simulink model "simulateur_1"  (R2022b)
settings: Solver=FixedStepAuto  StartTime=0.0  StopTime=10.0  FixedStep=dt  RelTol=1e-3
model workspace: external: MATLAB File /Users/antoine/Desktop/GPH/H2023/Design_2/simulation_équipe_1/init.m (data not in the file)
values from neighbouring files (symbols this model uses):
  dt = 0.000125    [init.m]
  f_1 = 100    [init.m]
  mode = 2    [init.m]
undefined symbols (not defined in the file or in its folder): magnitude
libraries: simulink x1, slpidlib x1, dspstat3 x1
settings Model: Creator=antoine  LastModifiedBy=antoine

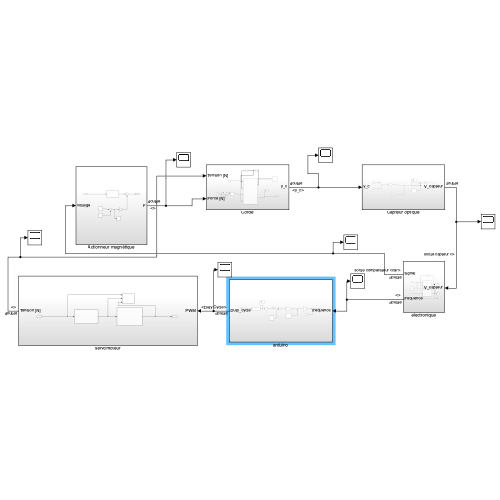
[thumbnail: Simulink's stored preview of the top-level diagram]
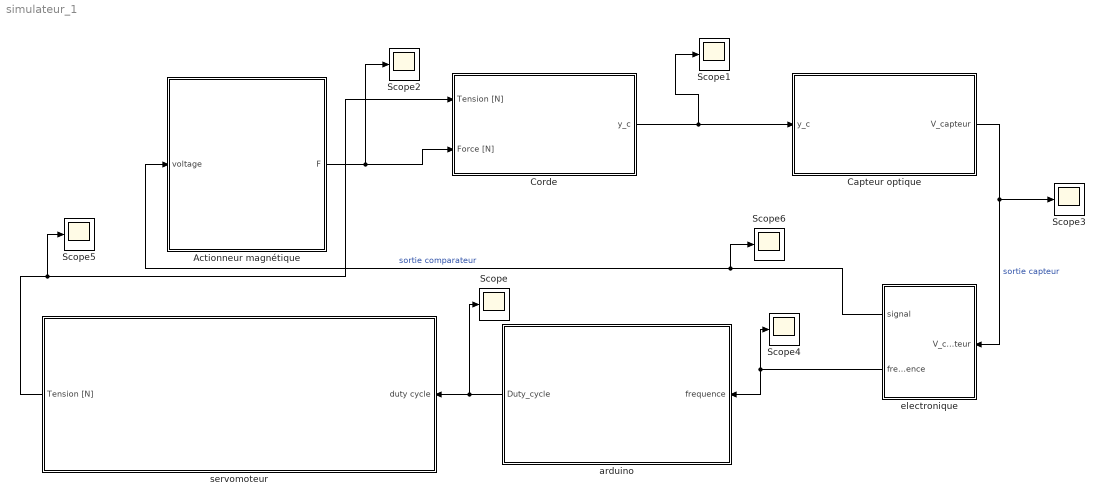
== system simulateur_1 ==
  Actionneur magnétique : Subsystem
  Capteur optique : Subsystem
  Corde : Subsystem
  Scope{,1..6} (7 alike) : Scope
  arduino : Subsystem
  electronique : Subsystem
  servomoteur : Subsystem
  wires:
  Corde/1(y_c) -> Capteur optique/1(y_c), Scope1/1
  Capteur optique/1(V_capteur) -> Scope3/1, electronique/1(V_capteur)  "sortie capteur"
  servomoteur/1(Tension [N]) -> Corde/1(Tension [N]), Scope5/1
  Actionneur magnétique/1(F) -> Scope2/1, Corde/2(Force [N])
  electronique/1(signal) -> Scope6/1, Actionneur magnétique/1(voltage)  "sortie comparateur"
  electronique/2(frequence) -> arduino/1(frequence), Scope4/1
  arduino/1(Duty_cycle) -> Scope/1, servomoteur/1(duty cycle)

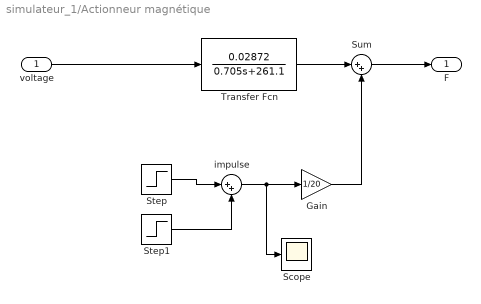
== system simulateur_1/Actionneur magnétique ==
  voltage : Inport
  Gain : Gain  Gain=1/20
  Scope : Scope
  Step : Step  Time=3*dt  SampleTime=0
  Step1 : Step  Time=6*dt  After=-1  SampleTime=0
  Sum : Sum  Inputs=|++
  Transfer Fcn : TransferFcn  Numerator=[0.02872]  Denominator=[0.705 261.1]
  impulse : Sum  Inputs=|++
  F : Outport
  wires:
  voltage/1 -> Transfer Fcn/1
  Transfer Fcn/1 -> Sum/1
  Sum/1 -> F/1
  Gain/1 -> Sum/2
  Step/1 -> impulse/1
  Step1/1 -> impulse/2
  impulse/1 -> Scope/1, Gain/1

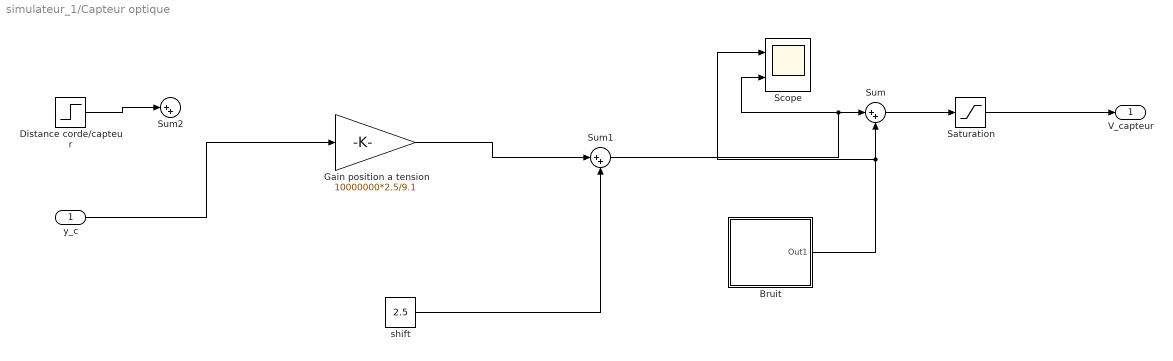
== system simulateur_1/Capteur optique ==
  y_c : Inport
  Bruit : Subsystem
  "Distance corde/capteur " : Step  Time=dt  After=0.00381  SampleTime=0
  Gain position a tension : Gain  Gain=10000000*2.5/9.1
  Saturation : Saturate  UpperLimit=5  LowerLimit=0
  Scope : Scope  NumInputPorts=2
  Sum : Sum  Inputs=|++
  Sum1 : Sum  Inputs=|++
  Sum2 : Sum  Inputs=|++
  shift : Constant  Value=2.5
  V_capteur : Outport
  wires:
  Sum/1 -> Saturation/1
  shift/1 -> Sum1/2
  Gain position a tension/1 -> Sum1/1
  Sum1/1 -> Scope/2, Sum/1
  Bruit/1(Out1) -> Scope/1, Sum/2
  Saturation/1 -> V_capteur/1
  "Distance corde/capteur "/1 -> Sum2/1
  y_c/1 -> Gain position a tension/1

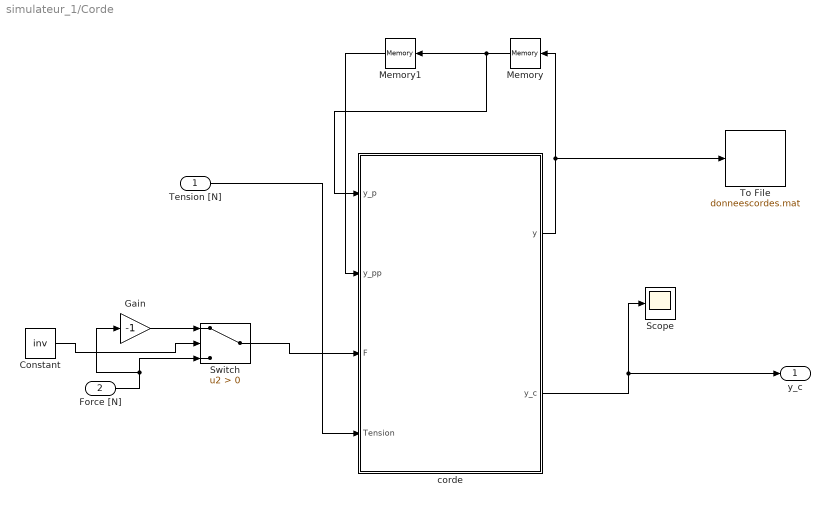
== system simulateur_1/Corde ==
  Tension [N] : Inport
  Force [N] : Inport  Port=2
  Constant : Constant  Value=inv
  Gain : Gain  Gain=-1
  Memory : Memory
  Memory1 : Memory
  Scope : Scope
  Switch : Switch  Criteria=u2 > Threshold  SaturateOnIntegerOverflow=off  InputSameDT=off
  To File : ToFile  Filename=donneescordes.mat  SaveFormat=Timeseries
  corde : MATLAB Function  TreatAsAtomicUnit=on
  y_c : Outport
  wires:
  corde/2(y_c) -> Scope/1, y_c/1
  Memory/1 -> corde/1(y_p), Memory1/1
  Memory1/1 -> corde/2(y_pp)
  corde/1(y) -> Memory/1, To File/1
  Switch/1 -> corde/3(F)
  Gain/1 -> Switch/1
  Force [N]/1 -> Switch/3, Gain/1
  Constant/1 -> Switch/2
  Tension [N]/1 -> corde/4(Tension)

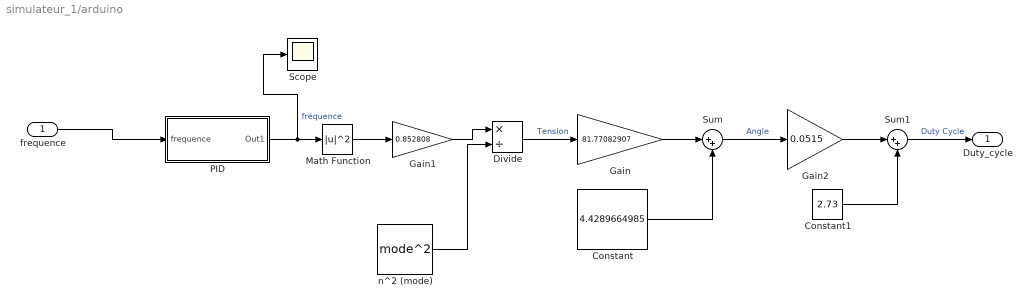
== system simulateur_1/arduino ==
  frequence : Inport
  Constant : Constant  Value=4.4289664985
  Constant1 : Constant  Value=2.73
  Divide : Product  Inputs=*/
  Gain : Gain  Gain=81.77082907
  Gain1 : Gain  Gain=0.852808
  Gain2 : Gain  Gain=0.0515
  Math Function : Math  Operator=magnitude^2
  PID : Subsystem
  Scope : Scope
  Sum : Sum  Inputs=|++
  Sum1 : Sum  Inputs=|++
  n^2 (mode) : Constant  Value=mode^2
  Duty_cycle : Outport
  wires:
  n^2 (mode)/1 -> Divide/2
  Gain1/1 -> Divide/1
  Gain2/1 -> Sum1/1
  Constant1/1 -> Sum1/2
  Divide/1 -> Gain/1  "Tension"
  Math Function/1 -> Gain1/1
  Gain/1 -> Sum/1
  PID/1(Out1) -> Scope/1, Math Function/1  "fréquence"
  Constant/1 -> Sum/2
  Sum1/1 -> Duty_cycle/1  "Duty Cycle"
  Sum/1 -> Gain2/1  "Angle"
  frequence/1 -> PID/1(frequence)

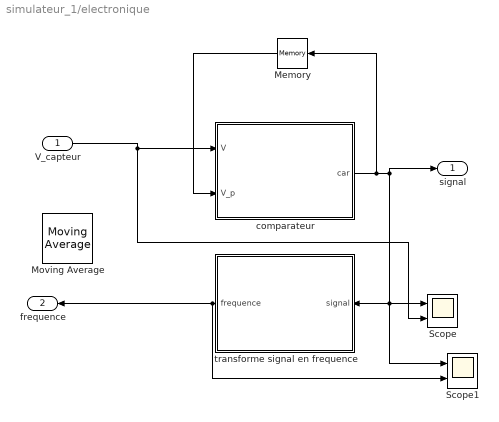
== system simulateur_1/electronique ==
  V_capteur : Inport
  Memory : Memory
  Moving Average : dspstat3/Moving Average  Method=Sliding window  ForgettingFactorPort=off  SpecifyWindowLength=on  WindowLength=10  OverlapLength=9  AllowArbitraryInputLength=off  ForgettingFactor=0.99  SimulateUsing=Interpreted execution
  Scope : Scope  NumInputPorts=2
  Scope1 : Scope  NumInputPorts=2
  comparateur : MATLAB Function  TreatAsAtomicUnit=on
  transforme signal en frequence : Subsystem
  signal : Outport
  frequence : Outport  Port=2
  wires:
  comparateur/1(car) -> Scope1/1, transforme signal en frequence/1(signal), Scope/1, signal/1, Memory/1
  Memory/1 -> comparateur/2(V_p)
  V_capteur/1 -> Scope/2, comparateur/1(V)
  transforme signal en frequence/1(frequence) -> Scope1/2, frequence/1

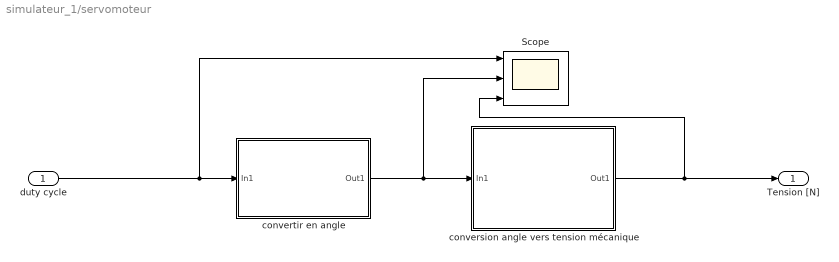
== system simulateur_1/servomoteur ==
  duty cycle : Inport
  Scope : Scope  NumInputPorts=3
  conversion angle vers tension mécanique : Subsystem
  convertir en angle : Subsystem
  Tension [N] : Outport
  wires:
  duty cycle/1 -> Scope/1, convertir en angle/1(In1)
  convertir en angle/1(Out1) -> Scope/2, conversion angle vers tension mécanique/1(In1)
  conversion angle vers tension mécanique/1(Out1) -> Scope/3, Tension [N]/1

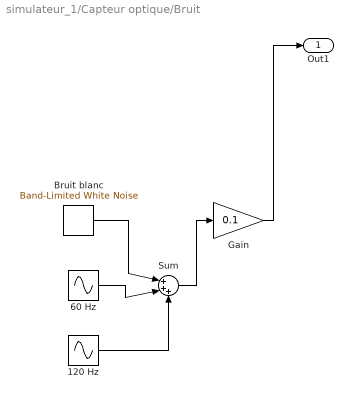
== system simulateur_1/Capteur optique/Bruit ==
  120 Hz : Sin  Frequency=120  SampleTime=0
  60 Hz : Sin  Frequency=60  SampleTime=0
  Bruit blanc : simulink/Sources/Band-Limited White Noise  Cov=[0.1]  Ts=0.1  seed=[23341]
  Gain : Gain  Gain=0.1
  Sum : Sum  Inputs=|+++
  Out1 : Outport
  wires:
  Bruit blanc/1 -> Sum/1
  60 Hz/1 -> Sum/2
  120 Hz/1 -> Sum/3
  Sum/1 -> Gain/1
  Gain/1 -> Out1/1

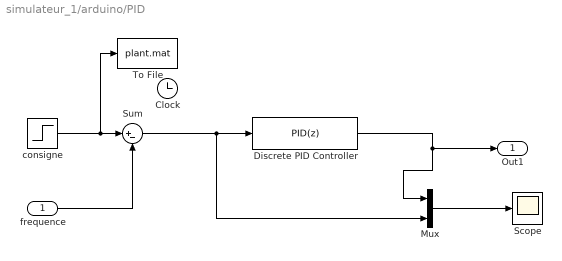
== system simulateur_1/arduino/PID ==
  frequence : Inport
  Clock : Clock
  Discrete PID Controller : slpidlib/PID Controller  Controller=PID  Form=Ideal  TimeDomain=Discrete-time  UseExternalTs=off  SampleTime=-1  IntegratorMethod=Trapezoidal  FilterMethod=Trapezoidal  ControllerParametersSource=internal  P=0.5  I=4.1  UseKiTs=off  D=0.4  N=10  UseFilter=on  TunerSelectOption=Transfer Function Based (PID Tuner App)  InitialConditionSource=internal  InitialConditionForIntegrator=0  InitialConditionForFilter=0  DifferentiatorICPrevScaledInput=0  ExternalReset=none  TrackingMode=off  Kt=1  LimitOutput=on  SatLimitsSource=internal  UpperSaturationLimit=1000  LowerSaturationLimit=-1000  LinearizeAsGain=off  AntiWindupMode=clamping  Kb=1  LimitIntegrator=on  UpperIntegratorSaturationLimit=1000  LowerIntegratorSaturationLimit=-1000  POutMin=[-1000]  POutMax=[1000]  IOutMin=[-1000]  IOutMax=[1000]  DOutMin=[-1000]  DOutMax=[1000]  NOutMin=[-1000]  NOutMax=[1000]  SumOutMin=[-1000]  SumOutMax=[1000]  SaturationOutMin=[]  SaturationOutMax=[]  PParamMin=[]  PParamMax=[]  IParamMin=[]  IParamMax=[]  DParamMin=[]  DParamMax=[]  NParamMin=[]  NParamMax=[]  KbParamMin=[]  KbParamMax=[]  KtParamMin=[]  KtParamMax=[]  KbOutMin=[]  KbOutMax=[]  KtOutMin=[]  KtOutMax=[]  IntegratorOutMin=[]  IntegratorOutMax=[]  FilterOutMin=[]  FilterOutMax=[]  SumI1OutMin=[]  SumI1OutMax=[]  SumI2OutMin=[]  SumI2OutMax=[]  SumI3OutMin=[]  SumI3OutMax=[]  SumI4OutMin=[]  SumI4OutMax=[]  SumDOutMin=[]  SumDOutMax=[]  DifferentiatorOutMin=[]  DifferentiatorOutMax=[]  FilterDiffOutCoefMin=[]  FilterDiffOutCoefMax=[]  ReciprocalOutMin=[]  ReciprocalOutMax=[]  SumDenOutMin=[]  SumDenOutMax=[]  SumNumOutMin=[]  SumNumOutMax=[]  DivideOutMin=[]  DivideOutMax=[]  UdiffTsProdOutMin=[]  UdiffTsProdOutMax=[]  NTsProdOutMin=[]  NTsProdOutMax=[]  UintegralTsProdOutMin=[]  UintegralTsProdOutMax=[]  UngainTsProdOutMin=[]  UngainTsProdOutMax=[]  ClampingZeroOutDataTypeStr=Inherit: Inherit via back propagation  ClampingZeroOutMin=[]  ClampingZeroOutMax=[]  FilterDenConstantOutDataTypeStr=Inherit: Inherit via back propagation  FilterDenConstantOutMin=[]  FilterDenConstantOutMax=[]  PCopyOutDataTypeStr=Inherit: Inherit via back propagation  PCopyOutMin=[]  PCopyOutMax=[]  NCopyOutDataTypeStr=Inherit: Inherit via back propagation  NCopyOutMin=[]  NCopyOutMax=[]  IntegratorContinuousStateAttributes=''  IntegratorStateMustResolveToSignalObject=off  IntegratorRTWStateStorageClass=Auto  FilterContinuousStateAttributes=''  FilterStateMustResolveToSignalObject=off  FilterRTWStateStorageClass=Auto  ParallelPVariant=Passthrough  IdealPVariant=InternalParameters  IVariant=InternalParameters  DVariant=InternalParameters  IntegratorVariant=Discrete  SatVariant=Enabled  AWVariant=DiscClampingIdeal  PCopyVariant=InternalParamsIdeal  TRVariant=Disabled  FdbkBlocksVariant=Feedback  IdealPFdbkVariant=InternalParameters  SatFdbkVariant=Passthrough  DerivativeFilterVariant=TrapezoidalFilter  NVariant=InternalParameters  NCopyVariant=InternalParameters  FilterICVariant=InternalICsFilter  IntegratorICVariant=InternalICs  ExternalResetVariant=Disabled  TRSumVariant=Passthrough  SumFdbkVariant=Enabled  SumVariant=Sum_PID  TsampFilterVariant=InternalTs  TsampNgainVariant=Passthrough  TsampIntegralVariant=Passthrough  ExternalSaturationOutDataTypeStr=Inherit: Same as second input
      settings: LibrarySourceBlock=simulink/Discrete/Discrete PID Controller
  Mux : Mux  Inputs=2
  Scope : Scope
  Sum : Sum  Inputs=|+-
  To File : ToFile  Filename=plant.mat  SaveFormat=Timeseries
  consigne : Step  Time=0  After=f_1  SampleTime=10
  Out1 : Outport
  wires:
  Mux/1 -> Scope/1
  consigne/1 -> To File/1, Sum/1
  frequence/1 -> Sum/2
  Sum/1 -> Discrete PID Controller/1, Mux/2
  Discrete PID Controller/1 -> Mux/1, Out1/1

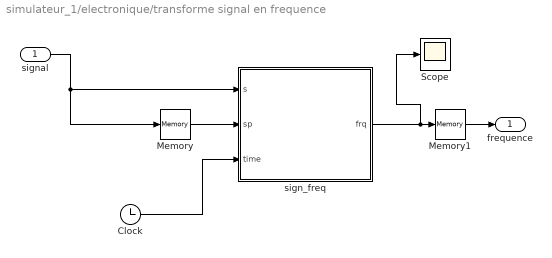
== system simulateur_1/electronique/transforme signal en frequence ==
  signal : Inport
  Clock : Clock
  Memory : Memory  InitialCondition=5
  Memory1 : Memory  InitialCondition=100
  Scope : Scope
  sign_freq : MATLAB Function  TreatAsAtomicUnit=on
  frequence : Outport
  wires:
  signal/1 -> Memory/1, sign_freq/1(s)
  sign_freq/1(frq) -> Memory1/1, Scope/1
  Clock/1 -> sign_freq/3(time)
  Memory/1 -> sign_freq/2(sp)
  Memory1/1 -> frequence/1

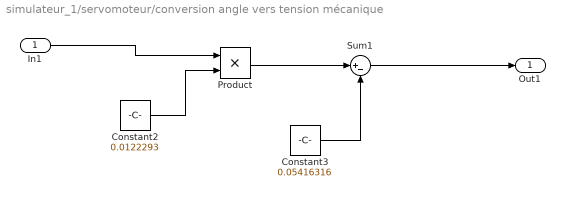
== system simulateur_1/servomoteur/conversion angle vers tension mécanique ==
  In1 : Inport
  Constant2 : Constant  Value=0.0122293
  Constant3 : Constant  Value=0.05416316
  Product : Product
  Sum1 : Sum  Inputs=|+-
  Out1 : Outport
  wires:
  Constant2/1 -> Product/2
  In1/1 -> Product/1
  Sum1/1 -> Out1/1
  Product/1 -> Sum1/1
  Constant3/1 -> Sum1/2

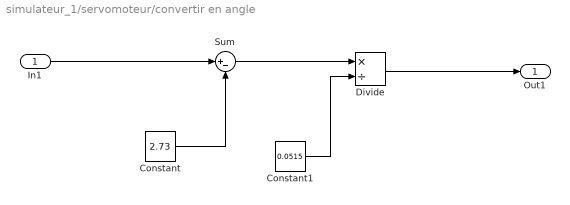
== system simulateur_1/servomoteur/convertir en angle ==
  In1 : Inport
  Constant : Constant  Value=2.73
  Constant1 : Constant  Value=0.0515
  Divide : Product  Inputs=*/
  Sum : Sum  Inputs=|+-
  Out1 : Outport
  wires:
  Divide/1 -> Out1/1
  Sum/1 -> Divide/1
  Constant/1 -> Sum/2
  In1/1 -> Sum/1
  Constant1/1 -> Divide/2

== matlab function simulateur_1/Corde/corde ==
  data: y output size=[1, n] [1..23]; y_p input size=[1, n]; y_pp input size=[1, n]; y_c output size=1; F input size=1; Tension input
function [y,y_c] = corde(y_p, y_pp,F,Tension)

dt = 0.000125;

f = 100; % [hz]
beta = 3.2 * 10^(-3);

mu = 7.68 * 10^(-3); % [kg/m]
masse = 0.004405; % [kg]s
Longueur = 0.44; % [m]
mu = masse/Longueur;
T_init = f^2 * 4 * Longueur^2 * mu/2;

if isempty(Tension)
    T = T_init;%f^2 * 4 * Longueur^2 * mu;%/mode^2; %f_1^2 * 4 * Longueur^2 * mu;
else
    T = Tension;
end
n = 21; % découper la corde en 'n' morceaux


p_actionneur = 16;
p_capteur = 5;

dx = Longueur/(n-1);

c = sqrt(complex(T)/(mu));


y = zeros(1,n);
f = zeros(1,n);
f(p_actionneur) = F;

for i = 2:(n - 1)
    pos = (y_p(i+1)-2*y_p(i)+y_p(i-1));
    first = (dt^2)/(mu + beta*dt);
    y(i) = first*(T*pos/dx^2 + mu*(2*y_p(i) - y_pp(i))/(dt^2) +beta*y_p(i)/dt +f(i));
end
y_c = y(p_capteur);


% Calcul constante de la simulation


end

== matlab function simulateur_1/electronique/comparateur ==
  data: V input; car output; V_p input
function car = comparateur(V, V_p)

if V <= 2
    car = 0;
elseif V >= 3
    car = 5;
else
    car = V_p;
end
end

== matlab function simulateur_1/electronique/transforme signal en frequence/sign_freq ==
  settings: updateMethod=DISCRETE
  data: s input; sp input; frq output; time input
function frq = sign_freq(s, sp, time)
persistent up_timer;
persistent down_timer;
% section pour pas avoir de bug
if isempty(up_timer)
    up_timer = 0;
end
if isempty(down_timer)
    down_timer = 0;
    frq = 100;
end
% pas de bug



if s == 5 && sp ~= 5 % debut du up
    up_timer = time;
elseif s == 0 && sp ~= 0 % debut du down
    down_timer = time;
end
period = abs((up_timer-down_timer)*2);
frq = 1/period;
